simulink model "gm_sampleModel1890_3_sub_sub"  (R2023a)
settings: Solver=VariableStepAuto  StartTime=0.0  StopTime=10.0  RelTol=1e-3
libraries: hdlsllib x2
settings Model: Creator=user1  LastModifiedBy=user1
settings OptimizationCC: BlockReduction=off  ConditionallyExecuteInputs=off
settings DebuggingCC: InheritedTsInSrcMsg=none

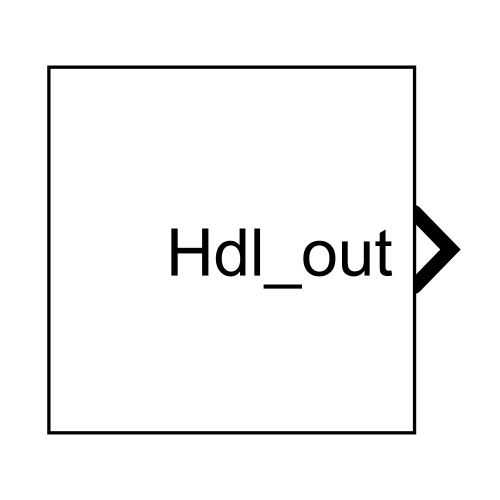
[thumbnail: Simulink's stored preview of the top-level diagram]
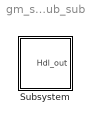
== system gm_sampleModel1890_3_sub_sub ==
  Subsystem : Subsystem

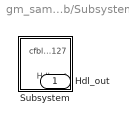
== system gm_sampleModel1890_3_sub_sub/Subsystem ==
  Subsystem : Subsystem
  Hdl_out : Outport  OutDataTypeStr=uint8

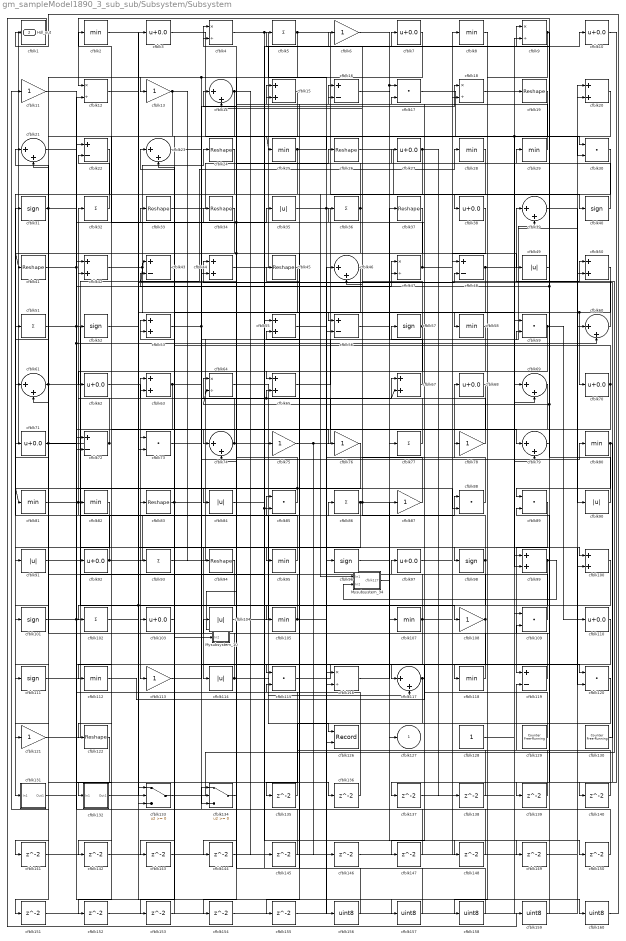
== system gm_sampleModel1890_3_sub_sub/Subsystem/Subsystem ==
  Mysubsystem_10 : Subsystem  TreatAsAtomicUnit=on  RTWFcnName=Mysubsystem_10
      settings: RTWFcnNameOpts=User specified  RTWFileNameOpts=Use function name
  Mysubsystem_34 : Subsystem  TreatAsAtomicUnit=on  RTWFcnName=Mysubsystem_34
      settings: RTWFcnNameOpts=User specified  RTWFileNameOpts=Use function name
  cfblk{1,5,32,36,51,77,86,93,102} (9 alike) : Sum  Inputs=+  OutDataTypeStr=uint8
  cfblk{3,7,10,27,38,62,68,70..71,92,97,103,110} (13 alike) : Bias  Bias=0.0  SaturateOnIntegerOverflow=off
  cfblk{15,20,42,44,50,53,55,63,65,67,99..100} (12 alike) : Sum  OutDataTypeStr=uint8
  cfblk{31,40,52,57,96,98,101,111} (8 alike) : Signum
  cfblk{35,49,84,90..91,104,114} (7 alike) : Abs  OutDataTypeStr=uint8  SaturateOnIntegerOverflow=off
  cfblk{2,8,25,28..29,58,80..82,95,105,107,112,118} (14 alike) : MinMax  OutDataTypeStr=uint8
  cfblk{6,11,13,75..76,78,87,108,113,121} (10 alike) : Gain  OutDataTypeStr=uint8
  cfblk{17,30,59,73,85,88..89,109,115,120} (10 alike) : DotProduct  OutDataTypeStr=uint8
  cfblk{4,9,12,18,47,64,116} (7 alike) : Product  Inputs=*/  OutDataTypeStr=uint8  RndMeth=Zero  SaturateOnIntegerOverflow=on
  cfblk{14,21,23,39,46,60..61,69,74,79,117} (11 alike) : Sum  Inputs=|++  OutDataTypeStr=uint8
  cfblk{16,22,43,48,56,72,119} (7 alike) : Sum  Inputs=+-  OutDataTypeStr=uint8
  cfblk{19,24,26,33..34,37,41,45,83,94,122} (11 alike) : Reshape
  cfblk126 : Record  FileSettingsInternal="{\"entries\":[{\"content\":{\"excelSettings\":{\"content\":{},\"type\":\"Streamout.ExcelSettings\"}},\"type\":\"Streamout.FileSettingStorage\",\"uuid\":\"\"}],\"packageUris\":[\"http:\\/\\/schema.mathworks.com\\/mf0\\/streamout_blocks\\/R2020a\"],\"version\":\"1.0\"}"  Layout=[1 1]  SignalsInternal="{\"entries\":[{\"content\":{\"signals\":[{\"content\":{\"blockPath\":[],\"dimensions\":[1],\"domain\":\"\",\"lineColor\":\"#a2142f\",\"plots\":[1],\"port\":1,\"signalID\":48435,\"signalName\":\"cfblk114\"},\"type\":\"RecordBlkView.Signal\",\"uuid\":\"\"},{\"content\":{\"blockPath\":[],\"dimensions\":[1],\"domain\":\"\",\"lineColor\":\"#139fff\",\"plots\":[1],\"port\":2,\"signalID\":48438,\"signalName\":\"cfblk117\"},\"type\":\"RecordBlkView.Signal\",\"uuid\":\"\"}]},\"type\":\"RecordBlkView.InputSignals\",\"uuid\":\"\"}],\"packageUris\":[\"http:\\/\\/schema.mathworks.com\\/mf0\\/streamout_blocks\\/R2020a\"],\"version\":\"1.0\"}"  VisualizationBindings="{\"xyplotplugin\":{\"info\":[{\"series\":[{\"bindingParametersList\":[{\"parameter\":\"X-Axis\",\"signalID\":48435,\"signalName\":\"cfblk114\"},{\"parameter\":\"Y-Axis\",\"signalID\":48438,\"signalName\":\"cfblk117\"}],\"seriesID\":18229}],\"subplotID\":1}]}}"  CompatibilityTag=XY  st=-1
  cfblk128 : Constant  OutDataTypeStr=uint8  SampleTime=-1
  cfblk129 : hdlsllib/Sources/Counter Free-Running  NumBits=16  tsamp=-1
  cfblk130 : hdlsllib/Sources/Counter Free-Running  NumBits=16  tsamp=-1
  cfblk131 : Subsystem
      settings: LibrarySourceBlock=|
      | hdlsllib/Ports &
      | Subsystems/Subsystem
  cfblk132 : Subsystem
      settings: LibrarySourceBlock=|
      | hdlsllib/Ports &
      | Subsystems/Subsystem
  cfblk133 : Switch  OutDataTypeStr=uint8  SaturateOnIntegerOverflow=off  InputSameDT=off
  cfblk134 : Switch  OutDataTypeStr=uint8  SaturateOnIntegerOverflow=off  InputSameDT=off
  cfblk{135..155} (21 alike) : Delay  SampleTime=1
  cfblk{156..160} (5 alike) : DataTypeConversion  OutDataTypeStr=uint8  SaturateOnIntegerOverflow=off  RndMeth=Floor
  cfblk127 : Outport  OutDataTypeStr=uint8  VectorParamsAs1DForOutWhenUnconnected=off
  Hdl_out : Outport  Port=2  OutDataTypeStr=uint8
  wires:
  cfblk42/1 -> cfblk79/2, cfblk24/1
  cfblk70/1 -> cfblk23/2, cfblk113/1
  cfblk14/1 -> cfblk145/1, cfblk21/2
  cfblk115/1 -> cfblk117/1
  cfblk29/1 -> cfblk13/1
  cfblk130/1 -> cfblk44/1
  cfblk111/1 -> cfblk28/1
  cfblk64/1 -> cfblk117/2
  cfblk5/1 -> cfblk144/1, cfblk38/1
  cfblk112/1 -> cfblk97/1
  cfblk74/1 -> cfblk33/1, cfblk98/1
  cfblk18/1 -> cfblk19/1
  cfblk81/1 -> cfblk82/1, cfblk108/1
  cfblk24/1 -> cfblk131/1(In1)
  cfblk89/1 -> cfblk119/1
  cfblk96/1 -> cfblk107/1
  cfblk49/1 -> cfblk12/1
  cfblk67/1 -> cfblk57/1
  cfblk36/1 -> cfblk16/2, cfblk4/2, cfblk41/1, Mysubsystem_10/1(In1)
  cfblk71/1 -> cfblk151/1, cfblk88/2
  cfblk133/1 -> cfblk39/1
  cfblk26/1 -> cfblk40/1
  cfblk121/1 -> cfblk85/1
  cfblk95/1 -> cfblk32/1
  cfblk33/1 -> cfblk26/1
  cfblk35/1 -> cfblk100/2, cfblk79/1
  cfblk75/1 -> cfblk146/1, cfblk67/1
  cfblk92/1 -> cfblk88/1, cfblk31/1
  cfblk80/1 -> cfblk140/1, cfblk139/1
  cfblk104/1 -> cfblk86/1
  cfblk79/1 -> cfblk9/1
  cfblk116/1 -> cfblk87/1
  cfblk85/1 -> cfblk43/2, cfblk81/1
  cfblk53/1 -> cfblk18/1, cfblk120/1
  cfblk4/1 -> cfblk96/1, cfblk150/1, cfblk85/2
  cfblk114/1 -> cfblk71/1, cfblk126/1
  cfblk62/1 -> cfblk83/1
  cfblk44/1 -> cfblk7/1
  cfblk109/1 -> cfblk63/1
  cfblk97/1 -> cfblk50/1
  cfblk2/1 -> cfblk133/1
  cfblk50/1 -> cfblk93/1, cfblk70/1
  cfblk83/1 -> cfblk59/2, Mysubsystem_10/2(In2)
  cfblk122/1 -> cfblk11/1
  cfblk86/1 -> cfblk133/2, cfblk149/1, cfblk6/1
  cfblk11/1 -> cfblk92/1
  cfblk7/1 -> cfblk134/2, cfblk101/1
  cfblk12/1 -> cfblk56/1
  cfblk56/1 -> cfblk100/1
  cfblk93/1 -> cfblk37/1
  cfblk45/1 -> cfblk103/1
  cfblk32/1 -> cfblk22/2
  cfblk132/1(Out1) -> cfblk48/2
  cfblk78/1 -> cfblk15/1
  cfblk38/1 -> cfblk61/1
  cfblk72/1 -> Hdl_out/1, cfblk42/2
  cfblk88/1 -> cfblk68/1
  cfblk99/1 -> cfblk118/1, Mysubsystem_34/2(In2)
  cfblk27/1 -> cfblk138/1, cfblk84/1
  cfblk87/1 -> cfblk46/2
  cfblk3/1 -> cfblk69/2
  cfblk105/1 -> cfblk51/1, cfblk78/1
  cfblk128/1 -> cfblk99/1
  cfblk61/1 -> cfblk21/1, cfblk120/2
  cfblk51/1 -> cfblk73/2, cfblk114/1
  cfblk129/1 -> cfblk36/1
  cfblk20/1 -> cfblk25/1, cfblk99/2
  cfblk84/1 -> cfblk10/1
  cfblk117/1 -> cfblk126/2, cfblk27/1
  cfblk41/1 -> cfblk160/1, cfblk12/2
  cfblk40/1 -> cfblk14/1
  cfblk101/1 -> cfblk75/1, cfblk60/2, cfblk47/2
  cfblk103/1 -> cfblk53/1
  cfblk37/1 -> cfblk65/1
  cfblk77/1 -> cfblk52/1
  cfblk6/1 -> cfblk148/1, cfblk17/1
  cfblk108/1 -> cfblk147/1, cfblk64/1
  cfblk16/1 -> cfblk77/1
  cfblk60/1 -> cfblk29/1
  cfblk82/1 -> cfblk111/1
  cfblk59/1 -> cfblk110/1, cfblk132/1(In1)
  cfblk65/1 -> cfblk39/2
  cfblk91/1 -> cfblk115/1
  cfblk48/1 -> cfblk56/2, cfblk20/1
  cfblk13/1 -> cfblk152/1, cfblk94/1
  cfblk100/1 -> cfblk105/1
  cfblk30/1 -> cfblk91/1
  cfblk15/1 -> cfblk73/1
  cfblk90/1 -> cfblk64/2, cfblk5/1, cfblk43/1
  cfblk39/1 -> cfblk90/1
  cfblk68/1 -> cfblk74/1
  cfblk63/1 -> cfblk47/1, cfblk102/1
  cfblk118/1 -> cfblk61/2
  cfblk134/1 -> cfblk104/1
  cfblk9/1 -> cfblk58/1, cfblk89/1
  cfblk57/1 -> cfblk14/2, cfblk74/2, cfblk17/2
  cfblk23/1 -> cfblk44/2
  cfblk19/1 -> cfblk62/1
  cfblk98/1 -> cfblk16/1, cfblk142/1, cfblk133/3
  cfblk25/1 -> cfblk122/1, cfblk30/1
  cfblk102/1 -> cfblk3/1
  cfblk22/1 -> cfblk72/2
  cfblk46/1 -> cfblk95/1
  cfblk113/1 -> cfblk80/1
  cfblk31/1 -> cfblk121/1, cfblk76/1
  cfblk47/1 -> cfblk49/1, cfblk2/1, cfblk4/1
  cfblk76/1 -> cfblk112/1
  cfblk73/1 -> cfblk67/2, cfblk65/2
  cfblk131/1(Out1) -> cfblk35/1
  cfblk119/1 -> cfblk45/1
  cfblk107/1 -> cfblk134/3, cfblk15/2, cfblk8/1
  cfblk69/1 -> cfblk116/2
  cfblk17/1 -> cfblk30/2
  cfblk120/1 -> cfblk135/1
  cfblk135/1 -> cfblk42/1
  cfblk21/1 -> cfblk136/1
  cfblk136/1 -> cfblk72/1
  cfblk10/1 -> cfblk137/1
  cfblk137/1 -> cfblk9/2
  cfblk138/1 -> cfblk115/2
  cfblk139/1 -> cfblk48/1
  cfblk140/1 -> cfblk119/2
  cfblk34/1 -> cfblk141/1
  cfblk141/1 -> cfblk109/1
  cfblk142/1 -> cfblk59/1
  cfblk43/1 -> cfblk143/1
  cfblk143/1 -> cfblk20/2
  cfblk144/1 -> cfblk18/2
  cfblk145/1 -> cfblk22/1
  cfblk146/1 -> cfblk50/2
  cfblk147/1 -> cfblk63/2
  cfblk148/1 -> cfblk134/1
  cfblk149/1 -> cfblk89/2
  cfblk150/1 -> cfblk23/1
  cfblk151/1 -> cfblk69/1
  cfblk152/1 -> cfblk60/1
  cfblk94/1 -> cfblk153/1
  cfblk153/1 -> cfblk53/2
  cfblk110/1 -> cfblk154/1
  cfblk154/1 -> cfblk46/1
  cfblk58/1 -> cfblk155/1
  cfblk155/1 -> cfblk116/1
  cfblk55/1 -> cfblk156/1
  cfblk156/1 -> cfblk34/1
  cfblk52/1 -> cfblk157/1
  cfblk157/1 -> cfblk55/1
  cfblk8/1 -> cfblk158/1
  cfblk158/1 -> cfblk55/2
  cfblk1/1 -> cfblk159/1
  cfblk159/1 -> cfblk109/2
  cfblk160/1 -> cfblk1/1
  cfblk28/1 -> Mysubsystem_34/1(In1)
  Mysubsystem_34/1(cfblk127) -> cfblk127/1

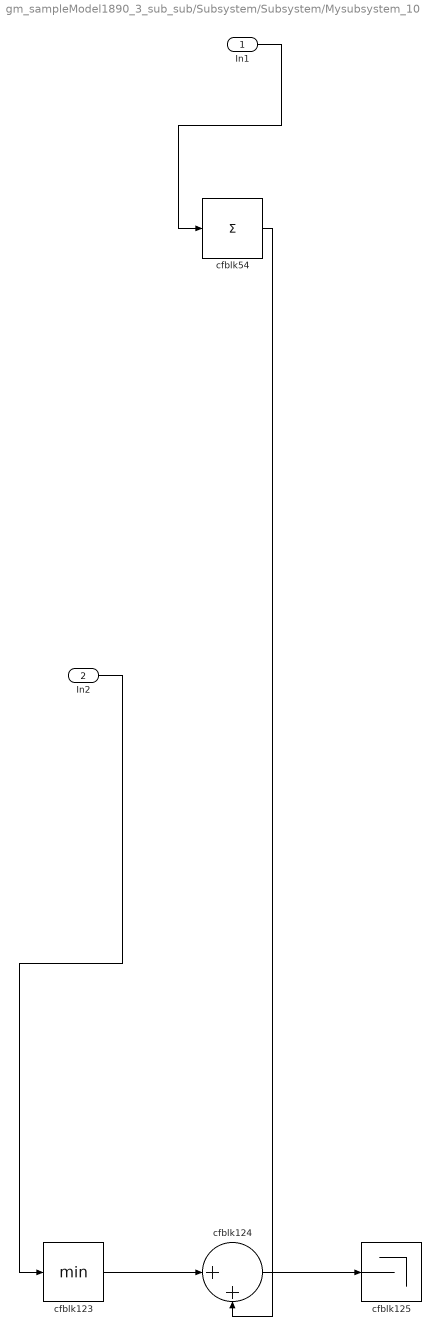
== system gm_sampleModel1890_3_sub_sub/Subsystem/Subsystem/Mysubsystem_10 ==
  In1 : Inport
  In2 : Inport  Port=2
  cfblk123 : MinMax
  cfblk124 : Sum  Inputs=|++
  cfblk125 : Terminator
  cfblk54 : Sum  Inputs=+
  wires:
  In2/1 -> cfblk123/1
  In1/1 -> cfblk54/1
  cfblk54/1 -> cfblk124/2
  cfblk124/1 -> cfblk125/1
  cfblk123/1 -> cfblk124/1

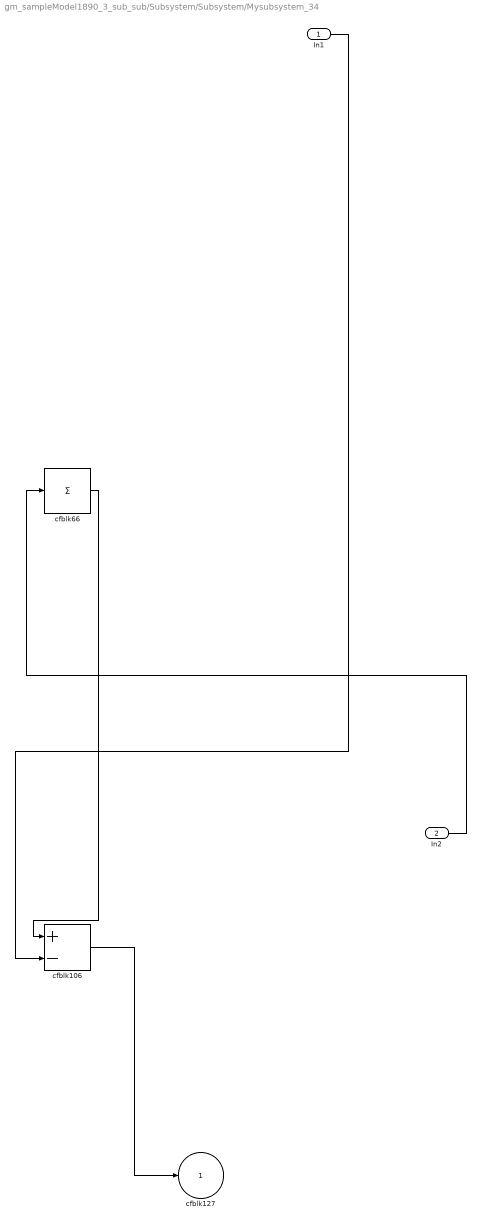
== system gm_sampleModel1890_3_sub_sub/Subsystem/Subsystem/Mysubsystem_34 ==
  In1 : Inport
  In2 : Inport  Port=2
  cfblk106 : Sum  Inputs=+-
  cfblk66 : Sum  Inputs=+
  cfblk127 : Outport  VectorParamsAs1DForOutWhenUnconnected=off
  wires:
  In1/1 -> cfblk106/2
  cfblk106/1 -> cfblk127/1
  cfblk66/1 -> cfblk106/1
  In2/1 -> cfblk66/1

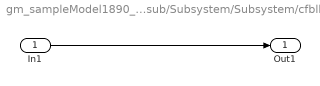
== system gm_sampleModel1890_3_sub_sub/Subsystem/Subsystem/cfblk131 ==
  In1 : Inport
  Out1 : Outport
  wires:
  In1/1 -> Out1/1

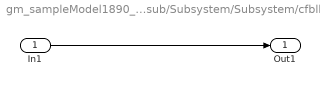
== system gm_sampleModel1890_3_sub_sub/Subsystem/Subsystem/cfblk132 ==
  In1 : Inport
  Out1 : Outport
  wires:
  In1/1 -> Out1/1
